simulink model "twist_filter_sl"  (R2018b)
settings: Solver=FixedStepDiscrete  StartTime=0.0  StopTime=inf  RelTol=1e-3
undefined symbols (not defined in the file): Header, Twist
libraries: robotlib x3
settings Model: Creator=keita  LastModifiedBy=keita
settings OptimizationCC: DefaultParameterBehavior=Inlined  UseDivisionForNetSlopeComputation=on  UseFloatMulNetSlope=on  InlineInvariantSignals=on  PassReuseOutputArgsAs=Individual arguments  ZeroExternalMemoryAtStartup=off  ZeroInternalMemoryAtStartup=off  NoFixptDivByZeroProtection=on  EfficientFloat2IntCast=on  LifeSpan=1  OptimizeBlockOrder=speed  DifferentSizesBufferReuse=on
settings DebuggingCC: ParameterTunabilityLossMsg=error  LibraryContextMissingDiagnostic=none
settings HardwareCC: ProdLongLongMode=on
settings SFSimCC: SimUseLocalCustomCode=off  MATLABDynamicMemAlloc=off
settings RTWCC: SystemTargetFile=ert.tlc  TemplateMakefile=ert_default_tmf  GenerateReport=on  RTWUseLocalCustomCode=off  IncludeHyperlinkInReport=on  LaunchReport=on  TargetLang=C++  GenerateTraceInfo=on  GenerateTraceReport=on  GenerateTraceReportSl=on  GenerateTraceReportSf=on  GenerateTraceReportEml=on
settings CodeAppCC: ForceParamTrailComments=on  IgnoreCustomStorageClasses=off  OperatorAnnotations=on  SimulinkDataObjDesc=on  SFDataObjDesc=on  CustomSymbolStrGlobalVar=rt$N$M  CustomSymbolStrType=$N$M  CustomSymbolStrFcn=$N$M$F  CustomSymbolStrMacro=$N$M  InsertBlockDesc=on
settings ERTTargetCC: TargetLangStandard=C++03 (ISO)  GenerateSampleERTMain=on  IncludeMdlTerminateFcn=off  CombineSignalStateStructs=on  SuppressErrorStatus=on  SupportAbsoluteTime=off  MultiInstanceERTCode=on  CodeInterfacePackaging=C++ class  SupportComplex=off  InlinedParameterPlacement=NonHierarchical  RootIOFormat=Structure reference  ERTCustomFileTemplate=example_file_process.tlc  ERTFilePackagingFormat=CompactWithDataFile

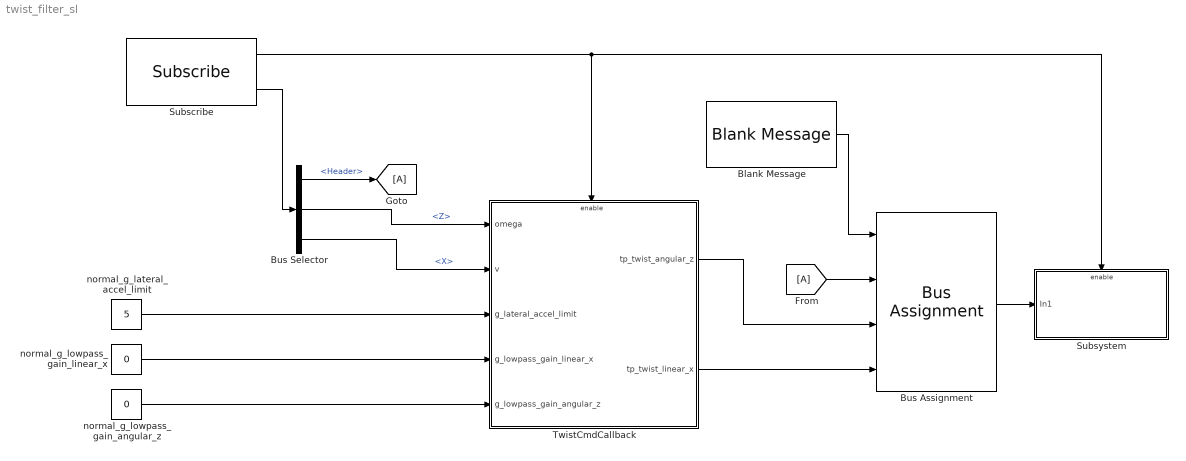
== system twist_filter_sl ==
  Blank Message : robotlib/Blank Message  messageClass=Message  entityType=geometry_msgs/TwistStamped  messageType=geometry_msgs/TwistStamped  SampleTime=inf
      settings: SourceProductBaseCode=RO
  Bus Assignment : BusAssignment  AssignedSignals=Header,Twist.Angular.Z,Twist.Linear.X
  Bus Selector : BusSelector  OutputSignals=Header,Twist.Angular.Z,Twist.Linear.X
  Subscribe : robotlib/Subscribe  topicSource=Select from ROS network  topic=/twist_raw  messageType=geometry_msgs/TwistStamped  sampleTime=-1  messageQueueLength=1
      settings: SourceProductBaseCode=RO
  Subsystem : Subsystem
  TwistCmdCallback : Subsystem
  normal_g_lateral_accel_limit : Constant  Value=5
  normal_g_lowpass_gain_angular_z : Constant  Value=0
  normal_g_lowpass_gain_linear_x : Constant  Value=0
  wires:
  TwistCmdCallback/2(tp_twist_linear_x) -> Bus Assignment/4
  Subscribe/2 -> Bus Selector/1
  Subscribe/1 -> TwistCmdCallback/Enable, Subsystem/Enable
  Blank Message/1 -> Bus Assignment/1
  Bus Selector/2 -> TwistCmdCallback/1(omega)  "<Z>"
  TwistCmdCallback/1(tp_twist_angular_z) -> Bus Assignment/3
  Bus Selector/3 -> TwistCmdCallback/2(v)  "<X>"
  normal_g_lateral_accel_limit/1 -> TwistCmdCallback/3(g_lateral_accel_limit)
  normal_g_lowpass_gain_linear_x/1 -> TwistCmdCallback/4(g_lowpass_gain_linear_x)
  normal_g_lowpass_gain_angular_z/1 -> TwistCmdCallback/5(g_lowpass_gain_angular_z)
  Bus Assignment/1 -> Subsystem/1(In1)
  Bus Selector/1 -> [A]  "<Header>"
  [A] -> Bus Assignment/2

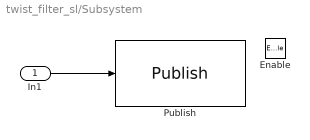
== system twist_filter_sl/Subsystem ==
  In1 : Inport
  Enable : EnablePort
  Publish : robotlib/Publish  topicSource=Select from ROS network  topic=/twist_cmd  messageType=geometry_msgs/TwistStamped  messageQueueLength=1
      settings: SourceProductBaseCode=RO
  wires:
  In1/1 -> Publish/1

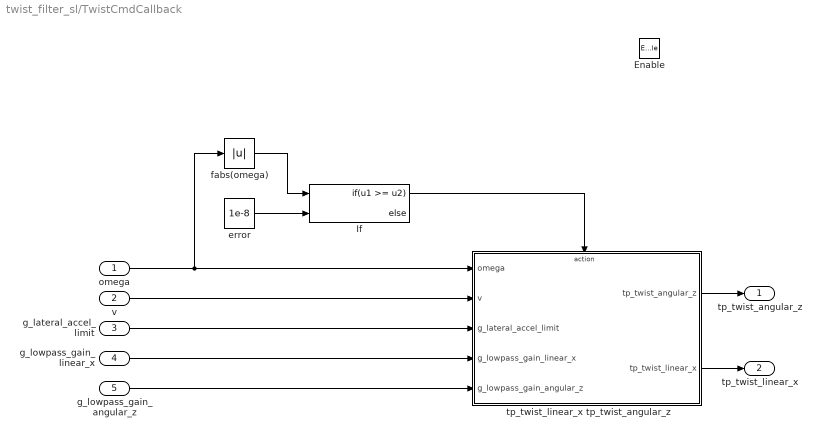
== system twist_filter_sl/TwistCmdCallback ==
  omega : Inport
  v : Inport  Port=2
  g_lateral_accel_limit : Inport  Port=3
  g_lowpass_gain_linear_x : Inport  Port=4
  g_lowpass_gain_angular_z : Inport  Port=5
  Enable : EnablePort
  If : If  NumInputs=2  IfExpression=u1 >= u2
  "error " : Constant  Value=1e-8
  fabs(omega) : Abs
  tp_twist_linear_x tp_twist_angular_z : Subsystem
  tp_twist_angular_z : Outport
  tp_twist_linear_x : Outport  Port=2
  wires:
  "error "/1 -> If/2
  tp_twist_linear_x tp_twist_angular_z/2(tp_twist_linear_x) -> tp_twist_linear_x/1
  tp_twist_linear_x tp_twist_angular_z/1(tp_twist_angular_z) -> tp_twist_angular_z/1
  v/1 -> tp_twist_linear_x tp_twist_angular_z/2(v)
  g_lateral_accel_limit/1 -> tp_twist_linear_x tp_twist_angular_z/3(g_lateral_accel_limit)
  g_lowpass_gain_linear_x/1 -> tp_twist_linear_x tp_twist_angular_z/4(g_lowpass_gain_linear_x)
  g_lowpass_gain_angular_z/1 -> tp_twist_linear_x tp_twist_angular_z/5(g_lowpass_gain_angular_z)
  fabs(omega)/1 -> If/1
  omega/1 -> tp_twist_linear_x tp_twist_angular_z/1(omega), fabs(omega)/1
  If/1 -> tp_twist_linear_x tp_twist_angular_z/Action

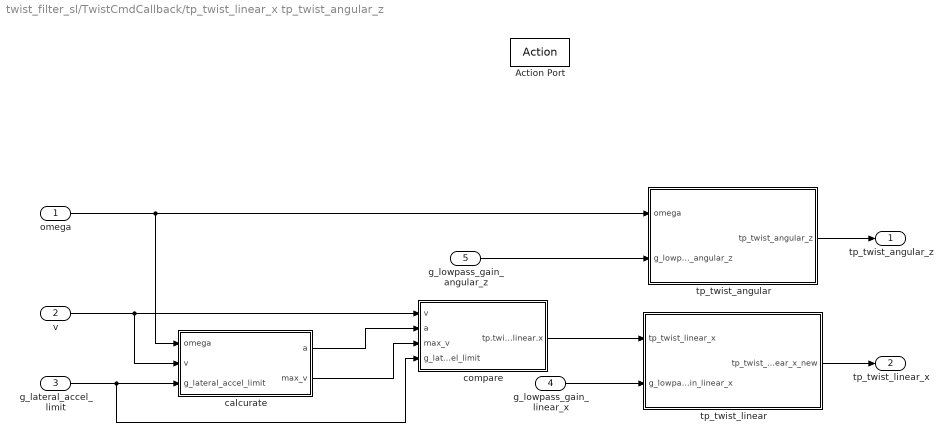
== system twist_filter_sl/TwistCmdCallback/tp_twist_linear_x tp_twist_angular_z ==
  omega : Inport
  v : Inport  Port=2
  g_lateral_accel_limit : Inport  Port=3
  g_lowpass_gain_linear_x : Inport  Port=4
  g_lowpass_gain_angular_z : Inport  Port=5
  Action Port : ActionPort  ActionType=then
  calcurate : Subsystem  TreatAsAtomicUnit=on
  "compare " : Subsystem
  tp_twist_angular : Subsystem
  tp_twist_linear : Subsystem
  tp_twist_angular_z : Outport
  tp_twist_linear_x : Outport  Port=2
  wires:
  v/1 -> calcurate/2(v), "compare "/1(v)
  tp_twist_linear/1(tp_twist_linear_x_new) -> tp_twist_linear_x/1
  "compare "/1(tp.twist.linear.x) -> tp_twist_linear/1(tp_twist_linear_x)
  calcurate/1(a) -> "compare "/2(a)
  calcurate/2(max_v) -> "compare "/3(max_v)
  g_lateral_accel_limit/1 -> "compare "/4(g_lateral_accel_limit), calcurate/3(g_lateral_accel_limit)
  tp_twist_angular/1(tp_twist_angular_z) -> tp_twist_angular_z/1
  omega/1 -> tp_twist_angular/1(omega), calcurate/1(omega)
  g_lowpass_gain_linear_x/1 -> tp_twist_linear/2(g_lowpass_gain_linear_x)
  g_lowpass_gain_angular_z/1 -> tp_twist_angular/2(g_lowpass_gain_angular_z)

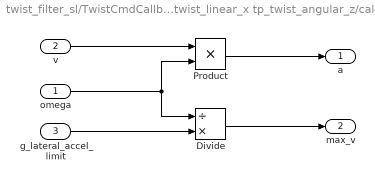
== system twist_filter_sl/TwistCmdCallback/tp_twist_linear_x tp_twist_angular_z/calcurate ==
  omega : Inport
  v : Inport  Port=2
  g_lateral_accel_limit : Inport  Port=3
  Divide : Product  Inputs=/*
  Product : Product
  a : Outport
  max_v : Outport  Port=2
  wires:
  Divide/1 -> max_v/1
  omega/1 -> Divide/1, Product/2
  v/1 -> Product/1
  Product/1 -> a/1
  g_lateral_accel_limit/1 -> Divide/2

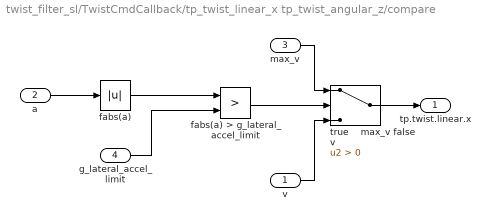
== system twist_filter_sl/TwistCmdCallback/tp_twist_linear_x tp_twist_angular_z/compare  ==
  v : Inport
  a : Inport  Port=2
  max_v : Inport  Port=3
  g_lateral_accel_limit : Inport  Port=4
  fabs(a) : Abs
  fabs(a) > g_lateral_accel_limit : RelationalOperator  Operator=>  OutDataTypeStr=boolean  RndMeth=Simplest
  "true    max_v false   v        " : Switch  Criteria=u2 > Threshold
  tp.twist.linear.x : Outport
  wires:
  g_lateral_accel_limit/1 -> fabs(a) > g_lateral_accel_limit/2
  fabs(a) > g_lateral_accel_limit/1 -> "true    max_v false   v        "/2
  fabs(a)/1 -> fabs(a) > g_lateral_accel_limit/1
  "true    max_v false   v        "/1 -> tp.twist.linear.x/1
  max_v/1 -> "true    max_v false   v        "/1
  a/1 -> fabs(a)/1
  v/1 -> "true    max_v false   v        "/3

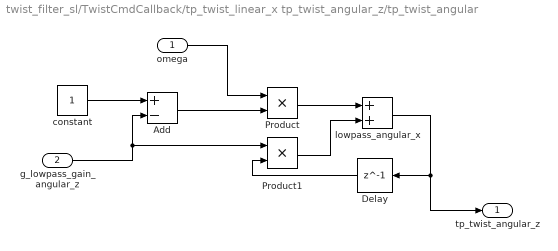
== system twist_filter_sl/TwistCmdCallback/tp_twist_linear_x tp_twist_angular_z/tp_twist_angular ==
  omega : Inport
  g_lowpass_gain_angular_z : Inport  Port=2
  Add : Sum  Inputs=+-
  Delay : Delay  DelayLength=1  InitialCondition=0
  Product : Product
  Product1 : Product
  constant : Constant
  lowpass_angular_x : Sum
  tp_twist_angular_z : Outport
  wires:
  lowpass_angular_x/1 -> tp_twist_angular_z/1, Delay/1
  g_lowpass_gain_angular_z/1 -> Add/2, Product1/1
  Product/1 -> lowpass_angular_x/1
  Add/1 -> Product/2
  Product1/1 -> lowpass_angular_x/2
  Delay/1 -> Product1/2
  constant/1 -> Add/1
  omega/1 -> Product/1

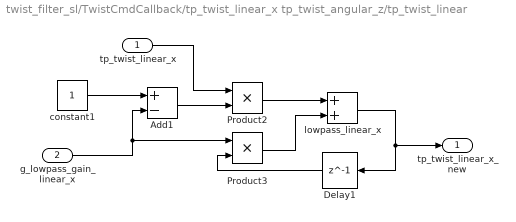
== system twist_filter_sl/TwistCmdCallback/tp_twist_linear_x tp_twist_angular_z/tp_twist_linear ==
  tp_twist_linear_x : Inport
  g_lowpass_gain_linear_x : Inport  Port=2
  Add1 : Sum  Inputs=+-
  Delay1 : Delay  DelayLength=1  InitialCondition=0
  Product2 : Product
  Product3 : Product
  constant1 : Constant
  lowpass_linear_x : Sum
  tp_twist_linear_x_new : Outport
  wires:
  Add1/1 -> Product2/2
  Delay1/1 -> Product3/2
  g_lowpass_gain_linear_x/1 -> Product3/1, Add1/2
  Product3/1 -> lowpass_linear_x/2
  lowpass_linear_x/1 -> tp_twist_linear_x_new/1, Delay1/1
  constant1/1 -> Add1/1
  Product2/1 -> lowpass_linear_x/1
  tp_twist_linear_x/1 -> Product2/1
